simulink model "worldGenerator"  (R2016b)
settings: Solver=FixedStepAuto  StartTime=0.0  StopTime=inf  RelTol=1e-3
model workspace (MAT data in the model file):
  SL_ROS_VariableLengthArrays_MaxSizes.CommonInfo.ArrayTruncateAction = 'EmitWarning'
  SL_ROS_VariableLengthArrays_MaxSizes.MsgTypeMap = containers.Map
  SL_ROS_VariableLengthArrays_MaxSizes.MsgTypeMap.serialization.keys = {'geometry_msgs/Polygon'}
  SL_ROS_VariableLengthArrays_MaxSizes.MsgTypeMap.serialization.values{1}.PropertyName = 'Points'
  SL_ROS_VariableLengthArrays_MaxSizes.MsgTypeMap.serialization.values{1}.DataType = 'geometry_msgs/Point32'
  SL_ROS_VariableLengthArrays_MaxSizes.MsgTypeMap.serialization.values{1}.MaxLength = 32
  SL_ROS_VariableLengthArrays_MaxSizes.MsgTypeMap.serialization.uniformity = 0
  SL_ROS_VariableLengthArrays_MaxSizes.MsgTypeMap.serialization.keyType = 'char'
  SL_ROS_VariableLengthArrays_MaxSizes.MsgTypeMap.serialization.valueType = 'any'
libraries: robotlib x2
(part 1 of 2)
settings Model: Creator=jupan  LastModifiedBy=jupan
settings OptimizationCC: MaxStackSize=64
settings DebuggingCC: ParameterTunabilityLossMsg=error  FcnCallInpInsideContextMsg=warning
settings HardwareCC: ProdBitPerPointer=32  ProdBitPerSizeT=32  ProdBitPerPtrDiffT=32  ProdLargestAtomicFloat=None  ProdIntDivRoundTo=Undefined  ProdEndianess=Unspecified  ProdWordSize=32  ProdHWDeviceType=Generic->Unspecified (assume 32-bit Generic)
settings RTWCC: SystemTargetFile=ert.tlc  HardwareBoard=Robot Operating System (ROS)  TLCOptions="-aInlineSetEventsForThisBaseRateFcn=TLC_FALSE -aSuppressMultiTaskScheduler=TLC_FALSE  -aRateBasedStepFcn=0"  TemplateMakefile=ert_default_tmf  Description=Embedded Coder  GenerateReport=on  Toolchain=Catkin  IncludeHyperlinkInReport=on  LaunchReport=on  TargetLang=C++  GenerateTraceInfo=on  GenerateTraceReport=on  GenerateTraceReportSl=on  GenerateTraceReportSf=on  GenerateTraceReportEml=on
settings CodeAppCC: ForceParamTrailComments=on  IgnoreCustomStorageClasses=off  OperatorAnnotations=on  SimulinkDataObjDesc=on  SFDataObjDesc=on  MATLABFcnDesc=on  InsertBlockDesc=on  MATLABSourceComments=on
settings ERTTargetCC: SupportVariableSizeSignals=on

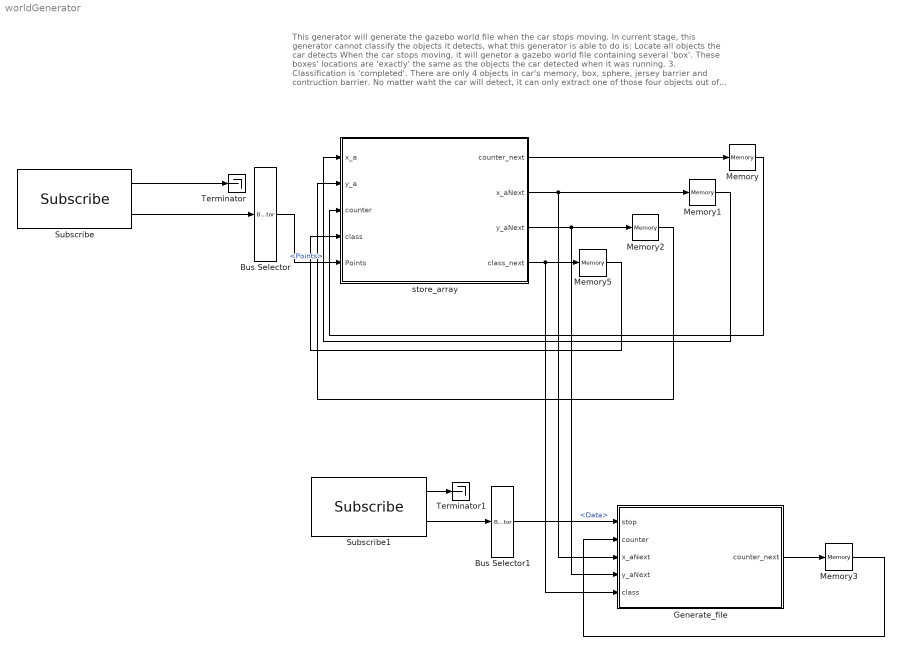
== system worldGenerator ==
  note: This generator will generate the gazebo world file when the car stops moving.
      | In current stage, this generator cannot classify the objects it detects, what this generator is able to do is:
      | Locate all objects the car detects
      | When the car stops moving, it will genetor a gazebo world file containing several 'box'.
      | These boxes' locations are 'exactly' the same as the objects the car detected when it was running.
      | 3. Classification is 'completed'. There are only 4 objects in car's memory, box, sphere, jersey barrier and contruction barrier. No matter waht the car will detect, it can only extract
      | one of those four objects out of its memory and put it into new world.
  Bus Selector : BusSelector  OutputSignals=Polygon.Points
  Bus Selector1 : BusSelector  OutputSignals=Data
  Generate_file : MATLAB Function  TreatAsAtomicUnit=on
  Memory{,1..3,5} (5 alike) : Memory
  Subscribe : robotlib/Subscribe  SourceLibraryInfo=This block requires Robotics System Toolbox  topicSource=Select from ROS network  topic=/detections  messageType=geometry_msgs/PolygonStamped  sampleTime=-1  messageQueueLength=1
  Subscribe1 : robotlib/Subscribe  SourceLibraryInfo=This block requires Robotics System Toolbox  topicSource=Specify your own  topic=/doIt  messageType=std_msgs/Bool  sampleTime=-1  messageQueueLength=1
  Terminator : Terminator
  Terminator1 : Terminator
  store_array : MATLAB Function  TreatAsAtomicUnit=on
  wires:
  Subscribe/1 -> Terminator/1
  Subscribe/2 -> Bus Selector/1
  Subscribe1/1 -> Terminator1/1
  Subscribe1/2 -> Bus Selector1/1
  store_array/1(counter_next) -> Memory/1
  store_array/2(x_aNext) -> Memory1/1, Generate_file/3(x_aNext)
  store_array/3(y_aNext) -> Memory2/1, Generate_file/4(y_aNext)
  Memory/1 -> store_array/3(counter)
  Memory1/1 -> store_array/1(x_a)
  Memory2/1 -> store_array/2(y_a)
  Bus Selector1/1 -> Generate_file/1(stop)  "<Data>"
  Generate_file/1(counter_next) -> Memory3/1
  Memory3/1 -> Generate_file/2(counter)
  store_array/4(class_next) -> Generate_file/5(class), Memory5/1
  Memory5/1 -> store_array/4(class)
  Bus Selector/1 -> store_array/5(Points)  "<Points>"

== matlab function worldGenerator/Generate_file ==
  data: stop input; counter_next output; counter input; x_aNext input; y_aNext input; class input
function counter_next = fcn(stop, counter, x_aNext, y_aNext, class)
%#codegen

if(stop && counter == 0)
    %'/home/jupan/cvchallenge_task3_ws/src/cvchallenge_task3/worlds/test.world'
    fid = fopen('gazebo_output.world', 'w+');
    % Fixed phase 1

    % <sdf version='1.4'>
    fprintf(fid, '<sdf version=''1.4''>\n');
    %   <world name='default'>
    fprintf(fid, '<world name=''default''>\n');
    %     <light name='sun' type='directional'>
    fprintf(fid, '<light name=''sun'' type=''directional''>\n');
    %       <cast_shadows>1</cast_shadows>
    fprintf(fid, '<cast_shadows>1</cast_shadows>\n');
    %       <pose>0 0 10 0 -0 0</pose>
    fprintf(fid, '<pose>0 0 10 0 -0 0</pose>\n');
    %       <diffuse>0.8 0.8 0.8 1</diffuse>
    fprintf(fid, '<diffuse>0.8 0.8 0.8 1</diffuse>\n');
    %       <specular>0.2 0.2 0.2 1</specular>
    fprintf(fid, '<specular>0.2 0.2 0.2 1</specular>\n');
    %       <attenuation>
    fprintf(fid, '<attenuation>\n');
    %         <range>1000</range>
    fprintf(fid, '<range>1000</range>\n');
    %         <constant>0.9</constant>
    fprintf(fid, '<constant>0.9</constant>\n');
    %         <linear>0.01</linear>
    fprintf(fid, '<linear>0.01</linear>\n');
    %         <quadratic>0.001</quadratic>
    fprintf(fid, '<quadratic>0.001</quadratic>\n');
    %       </attenuation>
    fprintf(fid, '</attenuation>\n');
    %       <direction>-0.5 0.1 -0.9</direction>
    fprintf(fid, '<direction>-0.5 0.1 -0.9</direction>\n');
    %     </light>
    fprintf(fid, '</light>\n');
    %     <model name='ground_plane'>
    fprintf(fid, '<model name=''ground_plane''>\n');
    %       <static>1</static>
    fprintf(fid, '<static>1</static>\n');
    %       <link name='link'>
    fprintf(fid, '<link name=''link''>\n');
    %         <collision name='collision'>
    fprintf(fid, '<collision name=''collision''>\n');
    %           <geometry>
    fprintf(fid, '<geometry>\n');
    %             <plane>
    fprintf(fid, '<plane>\n');
    %               <normal>0 0 1</normal>
    fprintf(fid, '<normal>0 0 1</normal>\n');
    %               <size>100 100</size>
    fprintf(fid, '<size>100 100</size>\n');
    %             </plane>
    fprintf(fid, '</plane>\n');
    %           </geometry>
    fprintf(fid, '</geometry>\n');
    %           <surface>
    fprintf(fid, '<surface>\n');
    %             <friction>
    fprintf(fid, '<friction>\n');
    %               <ode>
    fprintf(fid, '<ode>\n');
    %                 <mu>100</mu>
    fprintf(fid, '<mu>100</mu>\n');
    %                 <mu2>50</mu2>
    fprintf(fid, '<mu2>50</mu2>\n');
    %               </ode>
    fprintf(fid, '</ode>\n');
    %             </friction>
    fprintf(fid, '</friction>\n');
    %             <bounce/>
    fprintf(fid, '<bounce/>\n');
    %             <contact>
    fprintf(fid, '<contact>\n');
    %               <ode/>
    fprintf(fid, '<ode/>\n');
    %             </contact>
    fprintf(fid, '</contact>\n');
    %           </surface>
    fprintf(fid, '</surface>\n');
    %           <max_contacts>10</max_contacts>
    fprintf(fid, '<max_contacts>10</max_contacts>\n');
    %         </collision>
    fprintf(fid, '</collision>\n');
    %         <visual name='visual'>
    fprintf(fid, '<visual name=''visual''>\n');
    %           <cast_shadows>0</cast_shadows>
    fprintf(fid, '<cast_shadows>0</cast_shadows>\n');
    %           <geometry>
    fprintf(fid, '<geometry>\n');
    %             <plane>
    fprintf(fid, '<plane>\n');
    %               <normal>0 0 1</normal>
    fprintf(fid, '<normal>0 0 1</normal>\n');
    %               <size>100 100</size>
    fprintf(fid, '<size>100 100</size>\n');
    %             </plane>
    fprintf(fid, '</plane>\n');
    %           </geometry>
    fprintf(fid, '</geometry>\n');
    %           <material>
    fprintf(fid, '<material>\n');
    %             <script>
    fprintf(fid, '<script>\n');
    %               <uri>file://media/materials/scripts/gazebo.material</uri>
    fprintf(fid, '<uri>file://media/materials/scripts/gazebo.material</uri>\n');
    %               <name>Gazebo/Grey</name>
    fprintf(fid, '<name>Gazebo/Grey</name>\n');
    %             </script>
    fprintf(fid, '</script>\n');
    %           </material>
    fprintf(fid, '</material>\n');
    %         </visual>
    fprintf(fid, '</visual>\n');
    %         <velocity_decay>
    fprintf(fid, '<velocity_decay>\n');
    %           <linear>0</linear>
    fprintf(fid, '<linear>0</linear>\n');
    %           <angular>0</angular>
    fprintf(fid, '<angular>0</angular>\n');
    %         </velocity_decay>
    fprintf(fid, '</velocity_decay>\n');
    %         <self_collide>0</self_collide>
    fprintf(fid, '<self_collide>0</self_collide>\n');
    %         <kinematic>0</kinematic>
    fprintf(fid, '<kinematic>0</kinematic>\n');
    %         <gravity>1</gravity>
    fprintf(fid, '<gravity>1</gravity>\n');
    %       </link>
    fprintf(fid, '</link>\n');
    %     </model>
    fprintf(fid, '</model>\n');
    %     <physics type='ode'>
    fprintf(fid, '<physics type=''ode''>\n');
    %       <max_step_size>0.001</max_step_size>
    fprintf(fid, '<max_step_size>0.001</max_step_size>\n');
    %       <real_time_factor>1</real_time_factor>
    fprintf(fid, '<real_time_factor>1</real_time_factor>\n');
    %       <real_time_update_rate>1000</real_time_update_rate>
    fprintf(fid, '<real_time_update_rate>1000</real_time_update_rate>\n');
    %       <gravity>0 0 -9.8</gravity>
    fprintf(fid, '<gravity>0 0 -9.8</gravity>\n');
    %     </physics>
    fprintf(fid, '</physics>\n');
    %     <scene>
    fprintf(fid, '<scene>\n');
    %       <ambient>0.4 0.4 0.4 1</ambient>
    fprintf(fid, '<ambient>0.4 0.4 0.4 1</ambient>\n');
    %       <background>0.7 0.7 0.7 1</background>
    fprintf(fid, '<background>0.7 0.7 0.7 1</background>\n');
    %       <shadows>1</shadows>
    fprintf(fid, '<shadows>1</shadows>\n');
    %     </scene>
    fprintf(fid, '</scene>\n');
    %     <spherical_coordinates>
    fprintf(fid, '<spherical_coordinates>\n');
    %       <surface_model>EARTH_WGS84</surface_model>
    fprintf(fid, '<surface_model>EARTH_WGS84</surface_model>\n');
    %       <latitude_deg>0</latitude_deg>
    fprintf(fid, '<latitude_deg>0</latitude_deg>\n');
    %       <longitude_deg>0</longitude_deg>
    fprintf(fid, '<longitude_deg>0</longitude_deg>\n');
    %       <elevation>0</elevation>
    fprintf(fid, '<elevation>0</elevation>\n');
    %       <heading_deg>0</heading_deg>
    fprintf(fid, '<heading_deg>0</heading_deg>\n');
    %     </spherical_coordinates>
    fprintf(fid, '</spherical_coordinates>\n');
    %     <state world_name='default'>
    fprintf(fid, '<state world_name=''default''>\n');
    %       <sim_time>3437 164000000</sim_time>
    fprintf(fid, '<sim_time>3437 164000000</sim_time>\n');
    %       <real_time>3496 331503405</real_time>
    fprintf(fid, '<real_time>3496 331503405</real_time>\n');
    %       <wall_time>1490996669 500379643</wall_time>
    fprintf(fid, '<wall_time>1490996669 500379643</wall_time>\n');
    %       <model name='ground_plane'>
    fprintf(fid, '<model name=''ground_plane''>\n');
    %         <pose>0 0 0 0 -0 0</pose>
    fprintf(fid, '<pose>0 0 0 0 -0 0</pose>\n');
    %         <link name='link'>
    fprintf(fid, '<link name=''link''>\n');
    %           <pose>0 0 0 0 -0 0</pose>
    fprintf(fid, '<pose>0 0 0 0 -0 0</pose>\n');
    %           <velocity>0 0 0 0 -0 0</velocity>
    fprintf(fid, '<velocity>0 0 0 0 -0 0</velocity>\n');
    %           <acceleration>0 0 0 0 -0 0</acceleration>
    fprintf(fid, '<acceleration>0 0 0 0 -0 0</acceleration>\n');
    %           <wrench>0 0 0 0 -0 0</wrench>
    fprintf(fid, '<wrench>0 0 0 0 -0 0</wrench>\n');
    %         </link>
    fprintf(fid, '</link>\n');
    %       </model>
    fprintf(fid, '</model>\n');


    counter1 = 1;
    counter2 = 1;
    counter7 = 1;
    counter8 = 1;
    % First phase
    for i = 1:20
        if(x_aNext(i) ~= 0 && y_aNext(i) ~= 0)
            switch class(i)
              case 1 % unit_box
                  % <model name='unit_box_1'>
                  fprintf(fid, '<model name=''unit_box_');
                  fprintf(fid, '%d', int8(counter1));
                  fprintf(fid, '''>\n');
                  % <pose>-4 2 0.5 0 -0 0</pose>
                  fprintf(fid, ' <pose>');
                  fprintf(fid, '%f', x_aNext(i));fprintf(fid, ' ');
                  fprintf(fid, '%f', y_aNext(i));fprintf(fid, ' ');
                  fprintf(fid, '%f', 0.5);fprintf(fid, ' '); 
                  fprintf(fid, '%f', 0);fprintf(fid, ' ');
                  fprintf(fid, '-%f', 0);fprintf(fid, ' ');
                  fprintf(fid, '%f', 0);
                  fprintf(fid, '</pose>\n');
                  % <link name='link'>
                  fprintf(fid, ' <link name=''link''>\n');
                  % <pose>-4 2 0.5 0 -0 0</pose>
                  fprintf(fid, '  <pose>');
                  fprintf(fid, '%f', x_aNext(i));fprintf(fid, ' ');
                  fprintf(fid, '%f', y_aNext(i));fprintf(fid, ' ');
                  fprintf(fid, '%f', 0.5);fprintf(fid, ' '); 
                  fprintf(fid, '%f', 0);fprintf(fid, ' ');
                  fprintf(fid, '-%f', 0);fprintf(fid, ' ');
                  fprintf(fid, '%f', 0);
                  fprintf(fid, '</pose>\n');
                  % <velocity>0 0 0 0 -0 0</velocity>
                  fprintf(fid, '  <velocity>');
                  fprintf(fid, '%f', 0);fprintf(fid, ' ');
                  fprintf(fid, '%f', 0);fprintf(fid, ' ');
                  fprintf(fid, '%f', 0);fprintf(fid, ' '); 
                  fprintf(fid, '%f', 0);fprintf(fid, ' ');
                  fprintf(fid, '-%f', 0);fprintf(fid, ' ');
                  fprintf(fid, '%f', 0);
                  fprintf(fid, '</velocity>\n');
                  % <acceleration>0 0 0 0 -0 0</acceleration>
                  fprintf(fid, '  <acceleration>');
                  fprintf(fid, '%f', 0);fprintf(fid, ' ');
                  fprintf(fid, '%f', 0);fprintf(fid, ' ');
                  fprintf(fid, '%f', 0);fprintf(fid, ' '); 
                  fprintf(fid, '%f', 0);fprintf(fid, ' ');
                  fprintf(fid, '-%f', 0);fprintf(fid, ' ');
                  fprintf(fid, '%f', 0);
                  fprintf(fid, '</acceleration>\n');
                  % <wrench>0 0 0 0 -0 0</wrench>
                  fprintf(fid, '  <wrench>');
                  fprintf(fid, '%f', 0);fprintf(fid, ' ');
                  fprintf(fid, '%f', 0);fprintf(fid, ' ');
                  fprintf(fid, '%f', 0);fprintf(fid, ' '); 
                  fprintf(fid, '%f', 0);fprintf(fid, ' ');
                  fprintf(fid, '-%f', 0);fprintf(fid, ' ');
                  fprintf(fid, '%f', 0);
                  fprintf(fid, '</wrench>\n');
                  % </link>
                  fprintf(fid, ' </link>\n');
                  % </model>
                  fprintf(fid, '</model>\n');
                  counter1 = counter1 + 1;
              case 2 % unit_sphere
                  % <model name='unit_box_1'>
                  fprintf(fid, '<model name=''unit_sphere_');
                  fprintf(fid, '%d', int8(counter2));
                  fprintf(fid, '''>\n');
                  % <pose>-4 2 0.5 0 -0 0</pose>
                  fprintf(fid, ' <pose>');
                  fprintf(fid, '%f', x_aNext(i));fprintf(fid, ' ');
                  fprintf(fid, '%f', y_aNext(i));fprintf(fid, ' ');
                  fprintf(fid, '%f', 0.5);fprintf(fid, ' '); 
                  fprintf(fid, '%f', 0);fprintf(fid, ' ');
                  fprintf(fid, '-%f', 0);fprintf(fid, ' ');
                  fprintf(fid, '%f', 0);
                  fprintf(fid, '</pose>\n');
                  % <link name='link'>
                  fprintf(fid, ' <link name=''link''>\n');
                  % <pose>-4 2 0.5 0 -0 0</pose>
                  fprintf(fid, '  <pose>');
                  fprintf(fid, '%f', x_aNext(i));fprintf(fid, ' ');
                  fprintf(fid, '%f', y_aNext(i));fprintf(fid, ' ');
                  fprintf(fid, '%f', 0.5);fprintf(fid, ' '); 
                  fprintf(fid, '%f', 0);fprintf(fid, ' ');
                  fprintf(fid, '-%f', 0);fprintf(fid, ' ');
                  fprintf(fid, '%f', 0);
                  fprintf(fid, '</pose>\n');
                  % <velocity>0 0 0 0 -0 0</velocity>
                  fprintf(fid, '  <velocity>');
                  fprintf(fid, '%f', 0);fprintf(fid, ' ');
                  fprintf(fid, '%f', 0);fprintf(fid, ' ');
                  fprintf(fid, '%f', 0);fprintf(fid, ' '); 
                  fprintf(fid, '%f', 0);fprintf(fid, ' ');
                  fprintf(fid, '-%f', 0);fprintf(fid, ' ');
                  fprintf(fid, '%f', 0);
                  fprintf(fid, '</velocity>\n');
                  % <acceleration>0 0 0 0 -0 0</acceleration>
                  fprintf(fid, '  <acceleration>');
                  fprintf(fid, '%f', 0);fprintf(fid, ' ');
                  fprintf(fid, '%f', 0);fprintf(fid, ' ');
                  fprintf(fid, '%f', 0);fprintf(fid, ' '); 
                  fprintf(fid, '%f', 0);fprintf(fid, ' ');
                  fprintf(fid, '-%f', 0);fprintf(fid, ' ');
                  fprintf(fid, '%f', 0);
                  fprintf(fid, '</acceleration>\n');
                  % <wrench>0 0 0 0 -0 0</wrench>
                  fprintf(fid, '  <wrench>');
                  fprintf(fid, '%f', 0);fprintf(fid, ' ');
                  fprintf(fid, '%f', 0);fprintf(fid, ' ');
                  fprintf(fid, '%f', 0);fprintf(fid, ' '); 
                  fprintf(fid, '%f', 0);fprintf(fid, ' ');
                  fprintf(fid, '-%f', 0);fprintf(fid, ' ');
                  fprintf(fid, '%f', 0);
                  fprintf(fid, '</wrench>\n');
                  % </link>
                  fprintf(fid, ' </link>\n');
                  % </model>
                  fprintf(fid, '</model>\n');
                  counter2 = counter2 + 1;
                case 3
                    % <model name='unit_box_1'>
                  fprintf(fid, '<model name=''Construction Barrel_');
                  fprintf(fid, '%d', int8(counter7));
                  fprintf(fid, '''>\n');
                  % <pose>-4 2 0.5 0 -0 0</pose>
                  fprintf(fid, ' <pose>');
                  fprintf(fid, '%f', x_aNext(i));fprintf(fid, ' ');
                  fprintf(fid, '%f', y_aNext(i));fprintf(fid, ' ');
                  fprintf(fid, '%f', 0.5);fprintf(fid, ' '); 
                  fprintf(fid, '%f', 0);fprintf(fid, ' ');
                  fprintf(fid, '-%f', 0);fprintf(fid, ' ');
                  fprintf(fid, '%f', 0);
                  fprintf(fid, '</pose>\n');
                  % <link name='link'>
                  fprintf(fid, ' <link name=''link''>\n');
                  % <pose>-4 2 0.5 0 -0 0</pose>
                  fprintf(fid, '  <pose>');
                  fprintf(fid, '%f', x_aNext(i));fprintf(fid, ' ');
                  fprintf(fid, '%f', y_aNext(i));fprintf(fid, ' ');
                  fprintf(fid, '%f', 0.5);fprintf(fid, ' '); 
                  fprintf(fid, '%f', 0);fprintf(fid, ' ');
                  fprintf(fid, '-%f', 0);fprintf(fid, ' ');
                  fprintf(fid, '%f', 0);
                  fprintf(fid, '</pose>\n');
                  % <velocity>0 0 0 0 -0 0</velocity>
                  fprintf(fid, '  <velocity>');
                  fprintf(fid, '%f', 0);fprintf(fid, ' ');
                  fprintf(fid, '%f', 0);fprintf(fid, ' ');
                  fprintf(fid, '%f', 0);fprintf(fid, ' '); 
                  fprintf(fid, '%f', 0);fprintf(fid, ' ');
                  fprintf(fid, '-%f', 0);fprintf(fid, ' ');
                  fprintf(fid, '%f', 0);
                  fprintf(fid, '</velocity>\n');
                  % <acceleration>0 0 0 0 -0 0</acceleration>
                  fprintf(fid, '  <acceleration>');
                  fprintf(fid, '%f', 0);fprintf(fid, ' ');
                  fprintf(fid, '%f', 0);fprintf(fid, ' ');
                  fprintf(fid, '%f', 0);fprintf(fid, ' '); 
                  fprintf(fid, '%f', 0);fprintf(fid, ' ');
                  fprintf(fid, '-%f', 0);fprintf(fid, ' ');
                  fprintf(fid, '%f', 0);
                  fprintf(fid, '</acceleration>\n');
                  % <wrench>0 0 0 0 -0 0</wrench>
                  fprintf(fid, '  <wrench>');
                  fprintf(fid, '%f', 0);fprintf(fid, ' ');
                  fprintf(fid, '%f', 0);fprintf(fid, ' ');
                  fprintf(fid, '%f', 0);fprintf(fid, ' '); 
                  fprintf(fid, '%f', 0);fprintf(fid, ' ');
                  fprintf(fid, '-%f', 0);fprintf(fid, ' ');
                  fprintf(fid, '%f', 0);
                  fprintf(fid, '</wrench>\n');
                  % </link>
                  fprintf(fid, ' </link>\n');
                  % </model>
                  fprintf(fid, '</model>\n');
                  counter7 = counter7 + 1;
                case 4
                    % <model name='unit_box_1'>
                  fprintf(fid, '<model name=''jersey_barrier_');
                  fprintf(fid, '%d', int8(counter8));
                  fprintf(fid, '''>\n');
                  % <pose>-4 2 0.5 0 -0 0</pose>
                  fprintf(fid, ' <pose>');
                  fprintf(fid, '%f', x_aNext(i));fprintf(fid, ' ');
                  fprintf(fid, '%f', y_aNext(i));fprintf(fid, ' ');
                  fprintf(fid, '%f', 0.5);fprintf(fid, ' '); 
                  fprintf(fid, '%f', 0);fprintf(fid, ' ');
                  fprintf(fid, '-%f', 0);fprintf(fid, ' ');
                  fprintf(fid, '%f', 0);
                  fprintf(fid, '</pose>\n');
                  % <link name='link'>
                  fprintf(fid, ' <link name=''link''>\n');
                  % <pose>-4 2 0.5 0 -0 0</pose>
                  fprintf(fid, '  <pose>');
                  fprintf(fid, '%f', x_aNext(i));fprintf(fid, ' ');
                  fprintf(fid, '%f', y_aNext(i));fprintf(fid, ' ');
                  fprintf(fid, '%f', 0.5);fprintf(fid, ' '); 
                  fprintf(fid, '%f', 0);fprintf(fid, ' ');
                  fprintf(fid, '-%f', 0);fprintf(fid, ' ');
                  fprintf(fid, '%f', 0);
                  fprintf(fid, '</pose>\n');
                  % <velocity>0 0 0 0 -0 0</velocity>
                  fprintf(fid, '  <velocity>');
                  fprintf(fid, '%f', 0);fprintf(fid, ' ');
                  fprintf(fid, '%f', 0);fprintf(fid, ' ');
                  fprintf(fid, '%f', 0);fprintf(fid, ' '); 
                  fprintf(fid, '%f', 0);fprintf(fid, ' ');
                  fprintf(fid, '-%f', 0);fprintf(fid, ' ');
                  fprintf(fid, '%f', 0);
                  fprintf(fid, '</velocity>\n');
                  % <acceleration>0 0 0 0 -0 0</acceleration>
                  fprintf(fid, '  <acceleration>');
                  fprintf(fid, '%f', 0);fprintf(fid, ' ');
                  fprintf(fid, '%f', 0);fprintf(fid, ' ');
                  fprintf(fid, '%f', 0);fprintf(fid, ' '); 
                  fprintf(fid, '%f', 0);fprintf(fid, ' ');
                  fprintf(fid, '-%f', 0);fprintf(fid, ' ');
                  fprintf(fid, '%f', 0);
                  fprintf(fid, '</acceleration>\n');
                  % <wrench>0 0 0 0 -0 0</wrench>
                  fprintf(fid, '  <wrench>');
                  fprintf(fid, '%f', 0);fprintf(fid, ' ');
                  fprintf(fid, '%f', 0);fprintf(fid, ' ');
                  fprintf(fid, '%f', 0);fprintf(fid, ' '); 
                  fprintf(fid, '%f', 0);fprintf(fid, ' ');
                  fprintf(fid, '-%f', 0);fprintf(fid, ' ');
                  fprintf(fid, '%f', 0);
                  fprintf(fid, '</wrench>\n');
                  % </link>
                  fprintf(fid, ' </link>\n');
                  % </model>
                  fprintf(fid, '</model>\n');
                  counter8 = counter8 + 1;
              otherwise
                  disp('This class does not exist!') 
            end
        end
    end
    % </state>
    fprintf(fid, '</state>\n');

    counter3 = 1;
    counter4 = 1;
    counter5 = 1;
    counter6 = 1;
    % Second phase
    for j = 1:20
        if(x_aNext(j) ~= 0 && y_aNext(j) ~= 0)
            switch class(j)
              case 1 % unit_box
                  % <model name='unit_box_1'>
                  fprintf(fid, '<model name=''unit_box_');
                  fprintf(fid, '%d', int8(counter3));
                  fprintf(fid, '''>\n');
                  % <pose>-4 2 0.5 0 -0 0</pose>
                  fprintf(fid, ' <pose>');
                  fprintf(fid, '%f', x_aNext(j));fprintf(fid, ' ');
                  fprintf(fid, '%f', y_aNext(j));fprintf(fid, ' ');
                  fprintf(fid, '%f', 0.5);fprintf(fid, ' '); 
                  fprintf(fid, '%f', 0);fprintf(fid, ' ');
                  fprintf(fid, '-%f', 0);fprintf(fid, ' ');
                  fprintf(fid, '%f', 0);
                  fprintf(fid, '</pose>\n');
                  % <link name='link'>
                  fprintf(fid, ' <link name=''link''>\n');
                  % <inertial>
                  fprintf(fid, '  <inertial>\n');
                  % <mass>1</mass>
                  fprintf(fid, '   <mass>1</mass>\n');
                  % <inertia>
                  fprintf(fid, '   <inertia>\n');
                  % <ixx>1</ixx>
                  fprintf(fid, '    <ixx>1</ixx>\n');
                  fprintf(fid, '    <ixy>0</ixy>\n');
                  fprintf(fid, '    <ixz>0</ixz>\n');
                  fprintf(fid, '    <iyy>1</iyy>\n');
                  fprintf(fid, '    <iyz>0</iyz>\n');
                  fprintf(fid, '    <izz>1</izz>\n');
                  % </inertia>
                  fprintf(fid, '   </inertia>\n');
                  % </inertial>
                  fprintf(fid, '  </inertial>\n');
                  % <collision name='collision'>
                  fprintf(fid, '  <collision name=''collision''>\n');
                  % <geometry>
                  fprintf(fid, '   <geometry>\n');
                  % <box>
                  fprintf(fid, '    <box>\n');
                  % <size>1 1 1</size>
                  fprintf(fid, '     <size>');
                  fprintf(fid, '%d', int8(1));fprintf(fid, ' ');
                  fprintf(fid, '%d', int8(1));fprintf(fid, ' ');
                  fprintf(fid, '%d', int8(1));
                  fprintf(fid, '</size>\n');
                  % </box>
                  fprintf(fid, '    </box>\n');
                  % </geometry>
                  fprintf(fid, '   </geometry>\n');
                  % <max_contacts>10</max_contacts>
                  fprintf(fid, '   <max_contacts>10</max_contacts>\n');
                  % <surface>
                  fprintf(fid, '   <surface>\n');
                  % <bounce/>
                  fprintf(fid, '    <bounce/>\n');
                  % <friction>
                  fprintf(fid, '    <friction>\n');
                  % <ode/>
                  fprintf(fid, '     <ode/>\n');
                  % </friction>
                  fprintf(fid, '    </friction>\n');
                  % <contact>
                  fprintf(fid, '    <contact>\n');
                  % <ode/>
                  fprintf(fid, '     <ode/>\n');
                  % </contact>
                  fprintf(fid, '    </contact>\n');
                  % </surface>
                  fprintf(fid, '   </surface>\n');
                  % </collision>
                  fprintf(fid, '  </collision>\n');
                  % <visual name='visual'>
                  fprintf(fid, '  <visual name=''visual''>\n');
                  % <geometry>
                  fprintf(fid, '   <geometry>\n');
                  % <box>
                  fprintf(fid, '    <box>\n');
                  % <size>1 1 1</size>
                  fprintf(fid, '     <size>');
                  fprintf(fid, '%d', int8(1));fprintf(fid, ' ');
                  fprintf(fid, '%d', int8(1));fprintf(fid, ' ');
                  fprintf(fid, '%d', int8(1));
                  fprintf(fid, '</size>\n');
                  % </box>
                  fprintf(fid, '    </box>\n');
                  % </geometry>
                  fprintf(fid, '   </geometry>\n');
                  % <material>
                  fprintf(fid, '   <material>\n');
                  % <script>
                  fprintf(fid, '    <script>\n');
                  % <uri>file://media/materials/scripts/gazebo.material</uri>
                  fprintf(fid, '     <uri>file://media/materials/scripts/gazebo.material</uri>\n');
                  % <name>Gazebo/Grey</name>
                  fprintf(fid, '     <name>Gazebo/Grey</name>\n');
                  % </script>
                  fprintf(fid, '    </script>\n');
                  % </material>
                  fprintf(fid, '   </material>\n');
                  % </visual>
                  fprintf(fid, '  </visual>\n');
                  % <velocity_decay>
                  fprintf(fid, '  <velocity_decay>\n');
                  % <linear>0</linear>
                  fprintf(fid, '   <linear>0</linear>\n');
                  % <angular>0</angular>
                  fprintf(fid, '   <angular>0</angular>\n');
                  % </velocity_decay>
                  fprintf(fid, '  </velocity_decay>\n');
                  % <self_collide>0</self_collide>
                  fprintf(fid, '  <self_collide>0</self_collide>\n');
                  % <kinematic>0</kinematic>
                  fprintf(fid, '  <kinematic>0</kinematic>\n');
                  % <gravity>1</gravity>
                  fprintf(fid, '  <gravity>1</gravity>\n');
                  % </link>
                  fprintf(fid, ' </link>\n');
                  % <static>0</static>
                  fprintf(fid, ' <static>0</static>\n');
                  % </model>
                  fprintf(fid, '</model>\n');
                  counter3 = counter3 + 1;
              case 2 % unit_sphere
                  % <model name='unit_sphere_1'>
                  fprintf(fid, '<model name=''unit_sphere_');
                  fprintf(fid, '%d', int8(counter4));
                  fprintf(fid, '''>\n');
                  % <pose>-4 2 0.5 0 -0 0</pose>
                  fprintf(fid, ' <pose>');
                  fprintf(fid, '%f', x_aNext(j));fprintf(fid, ' ');
                  fprintf(fid, '%f', y_aNext(j));fprintf(fid, ' ');
                  fprintf(fid, '%f', 0.5);fprintf(fid, ' '); 
                  fprintf(fid, '%f', 0);fprintf(fid, ' ');
                  fprintf(fid, '-%f', 0);fprintf(fid, ' ');
                  fprintf(fid, '%f', 0);
                  fprintf(fid, '</pose>\n');
                  % <link name='link'>
                  fprintf(fid, ' <link name=''link''>\n');
                  % <inertial>
                  fprintf(fid, '  <inertial>\n');
                  % <mass>1</mass>
                  fprintf(fid, '   <mass>1</mass>\n');
                  % <inertia>
                  fprintf(fid, '   <inertia>\n');
                  % <ixx>1</ixx>
                  fprintf(fid, '    <ixx>1</ixx>\n');
                  fprintf(fid, '    <ixy>0</ixy>\n');
                  fprintf(fid, '    <ixz>0</ixz>\n');
                  fprintf(fid, '    <iyy>1</iyy>\n');
                  fprintf(fid, '    <iyz>0</iyz>\n');
                  fprintf(fid, '    <izz>1</izz>\n');
                  % </inertia>
                  fprintf(fid, '   </inertia>\n');
                  % </inertial>
                  fprintf(fid, '  </inertial>\n');
                  % <collision name='collision'>
                  fprintf(fid, '  <collision name=''collision''>\n');
                  % <geometry>
                  fprintf(fid, '   <geometry>\n');
                  % <box>
                  fprintf(fid, '    <sphere>\n');
                  % <size>1 1 1</size>
                  fprintf(fid, '    <radius>0.5</radius>\n');
                  % </box>
                  fprintf(fid, '    </sphere>\n');
                  % </geometry>
                  fprintf(fid, '   </geometry>\n');
                  % <max_contacts>10</max_contacts>
                  fprintf(fid, '   <max_contacts>10</max_contacts>\n');
                  % <surface>
                  fprintf(fid, '   <surface>\n');
                  % <bounce/>
                  fprintf(fid, '    <bounce/>\n');
                  % <friction>
                  fprintf(fid, '    <friction>\n');
                  % <ode/>
                  fprintf(fid, '     <ode/>\n');
                  % </friction>
                  fprintf(fid, '    </friction>\n');
                  % <contact>
                  fprintf(fid, '    <contact>\n');
                  % <ode/>
                  fprintf(fid, '     <ode/>\n');
                  % </contact>
                  fprintf(fid, '    </contact>\n');
                  % </surface>
                  fprintf(fid, '   </surface>\n');
                  % </collision>
                  fprintf(fid, '  </collision>\n');
                  % <visual name='visual'>
                  fprintf(fid, '  <visual name=''visual''>\n');
                  % <geometry>
                  fprintf(fid, '   <geometry>\n');
                  % <sphere>
                  fprintf(fid, '    <sphere>\n');
                  % <radius>0.5</radius>
                  fprintf(fid, '     <radius>0.5</radius>\n');
                  % </sphere>
                  fprintf(fid, '    </sphere>\n');
                  % </geometry>
                  fprintf(fid, '   </geometry>\n');
                  % <material>
                  fprintf(fid, '   <material>\n');
                  % <script>
                  fprintf(fid, '    <script>\n');
                  % <uri>file://media/materials/scripts/gazebo.material</uri>
                  fprintf(fid, '     <uri>file://media/materials/scripts/gazebo.material</uri>\n');
                  % <name>Gazebo/Grey</name>
                  fprintf(fid, '     <name>Gazebo/Grey</name>\n');
                  % </script>
                  fprintf(fid, '    </script>\n');
                  % </material>
                  fprintf(fid, '   </material>\n');
                  % </visual>
                  fprintf(fid, '  </visual>\n');
                  % <velocity_decay>
                  fprintf(fid, '  <velocity_decay>\n');
                  % <linear>0</linear>
                  fprintf(fid, '   <linear>0</linear>\n');
                  % <angular>0</angular>
                  fprintf(fid, '   <angular>0</angular>\n');
                  % </velocity_decay>
                  fprintf(fid, '  </velocity_decay>\n');
                  % <self_collide>0</self_collide>
                  fprintf(fid, '  <self_collide>0</self_collide>\n');
                  % <kinematic>0</kinematic>
                  fprintf(fid, '  <kinematic>0</kinematic>\n');
                  % <gravity>1</gravity>
                  fprintf(fid, '  <gravity>1</gravity>\n');
                  % </link>
                  fprintf(fid, ' </link>\n');
                  % <static>0</static>
                  fprintf(fid, ' <static>0</static>\n');
                  % </model>
                  fprintf(fid, '</model>\n');
                  counter4 = counter4 + 1;
                case 3
                    % Construction Barrel
                    fprintf(fid, '<model name=''Construction Barrel_');
                              fprintf(fid, '%d', int8(counter5));
                              fprintf(fid, '''>\n');
                    fprintf(fid, ['<link name=''link''>\n'...
                            ,'<inertial>\n'...
                             , '<pose>0 0 0.4 0 -0 0</pose>\n'...
                              ,'<mass>500</mass>\n'...
                              ,'<inertia>\n'...
                                ,'<ixx>51.2096</ixx>\n'...
                                ,'<iyy>51.2096</iyy>\n'...
                                ,'<izz>25</izz>\n'...
                                ,'<ixy>0</ixy>\n'...
                                ,'<ixz>0</ixz>\n'...
                                ,'<iyz>0</iyz>\n'...
                              ,'</inertia>\n'...
                            ,'</inertial>\n'...
                            ,'<collision name=''collision''>\n'...
                              ,'<geometry>\n'...
                                ,'<mesh>\n'...
                                  ,'<uri>model://construction_barrel/meshes/construction_barrel.dae</uri>\n'...
                                ,'</mesh>\n'...
                              ,'</geometry>\n'...
                              ,'<max_contacts>10</max_contacts>\n'...
                              ,'<surface>\n'...
                                ,'<bounce/>\n'...
                                ,'<friction>\n'...
                                  ,'<ode/>\n'...
                                ,'</friction>\n'...
                                ,'<contact>\n'...
                                  ,'<ode/>\n'...
                                ,'</contact>\n'...
                              ,'</surface>\n'...
                            ,'</collision>\n'...
                            ,'<visual name=''visual''>\n'...
                              ,'<geometry>\n'...
                                ,'<mesh>\n'...
                                  ,'<uri>model://construction_barrel/meshes/construction_barrel.dae</uri>\n'...
                                ,'</mesh>\n'...
                              ,'</geometry>\n'...
                            ,'</visual>\n'...
                            ,'<velocity_decay>\n'...
                              ,'<linear>0</linear>\n'...
                              ,'<angular>0</angular>\n'...
                            ,'</velocity_decay>\n'...
                            ,'<self_collide>0</self_collide>\n'...
                            ,'<kinematic>0</kinematic>\n'...
                            ,'<gravity>1</gravity>\n'...
                          ,'</link>\n']);
                      fprintf(fid, ' <pose>');
                          fprintf(fid, '%f', x_aNext(j));fprintf(fid, ' ');
                          fprintf(fid, '%f', y_aNext(j));fprintf(fid, ' ');
                          fprintf(fid, '%f', 0.5);fprintf(fid, ' '); 
                          fprintf(fid, '%f', 0);fprintf(fid, ' ');
                          fprintf(fid, '-%f', 0);fprintf(fid, ' ');
                          fprintf(fid, '%f', 0);
                          fprintf(fid, '</pose>\n');
                     fprintf(fid, ['<static>0</static>\n'...
                    ,'</model>\n']);
                     counter5 = counter5 + 1;
                case 4
                    % jersey barrier
                    fprintf(fid, '<model name=''jersey_barrier_');
                              fprintf(fid, '%d', int8(counter6));
                              fprintf(fid, '''>\n');
                    fprintf(fid, ['<static>1</static>\n'...
                          ,'<link name=''link''>\n'...
                            ,'<visual name=''visual''>\n'...
                             ,'<geometry>\n'...
                                ,'<mesh>\n'...
                                  ,'<uri>model://jersey_barrier/meshes/jersey_barrier.dae</uri>\n'...
                                ,'</mesh>\n'...
                              ,'</geometry>\n'...
                            ,'</visual>\n'...
                            ,'<collision name=''upright''>\n'...
                              ,'<pose>0 0 0.5715 0 -0 0</pose>\n'...
                              ,'<geometry>\n'...
                                ,'<box>\n'...
                                  ,'<size>4.06542 0.3063 1.143</size>\n'...
                                ,'</box>\n'...
                              ,'</geometry>\n'...
                              ,'<max_contacts>10</max_contacts>\n'...
                              ,'<surface>\n'...
                                ,'<bounce/>\n'...
                                ,'<friction>\n'...
                                  ,'<ode/>\n'...
                                ,'</friction>\n'...
                                ,'<contact>\n'...
                                  ,'<ode/>\n'...
                                ,'</contact>\n'...
                              ,'</surface>\n'...
                            ,'</collision>\n'...
                            ,'<collision name=''base''>\n'...
                              ,'<pose>0 0 0.032258 0 -0 0</pose>\n'...
                              ,'<geometry>\n'...
                                ,'<box>\n'...
                                  ,'<size>4.06542 0.8107 0.064516</size>\n'...
                                ,'</box>\n'...
                              ,'</geometry>\n'...
                              ,'<max_contacts>10</max_contacts>\n'...
                              ,'<surface>\n'...
                                ,'<bounce/>\n'...
                                ,'<friction>\n'...
                                  ,'<ode/>\n'...
                                ,'</friction>\n'...
                                ,'<contact>\n'...
                                  ,'<ode/>\n'...
                                ,'</contact>\n'...
                              ,'</surface>\n'...
                            ,'</collision>\n'...
                            ,'<collision name=''base2''>\n'...
                              ,'<pose>0 0 0.1 0 -0 0</pose>\n'...
                              ,'<geometry>\n'...
                                ,'<box>\n'...
                                  ,'<size>4.06542 0.65 0.1</size>\n'...
                                ,'</box>\n'...
                              ,'</geometry>\n'...
                              ,'<max_contacts>10</max_contacts>\n'...
                              ,'<surface>\n'...
                                ,'<bounce/>\n'...
                                ,'<friction>\n'...
                                  ,'<ode/>\n'...
                                ,'</friction>\n'...
                                ,'<contact>\n'...
                                  ,'<ode/>\n'...
                                ,'</contact>\n'...
                              ,'</surface>\n'...
                            ,'</collision>\n'...
                            ,'<collision name=''base3''>\n'...
                              ,'<pose>0 0 0.2 0 -0 0</pose>\n'...
                              ,'<geometry>\n'...
                                ,'<box>\n'...
                                  ,'<size>4.06542 0.5 0.1</size>\n'...
                                ,'</box>\n'...
                              ,'</geometry>\n'...
                              ,'<max_contacts>10</max_contacts>\n'...
                              ,'<surface>\n'...
                                ,'<bounce/>\n'...
                                ,'<friction>\n'...
                                  ,'<ode/>\n'...
                                ,'</friction>\n'...
                                ,'<contact>\n'...
                                  ,'<ode/>\n'...
                                ,'</contact>\n'...
                              ,'</surface>\n'...
                            ,'</collision>\n'...
                            ,'<collision name=''left-angle''>\n'...
                              ,'<pose>0 -0.224 0.2401 0.9 -0 0</pose>\n'...
                              ,'<geometry>\n'...
                                ,'<box>\n'...
                                  ,'<size>4.06542 0.5 0.064516</size>\n'...
                                ,'</box>\n'...
                              ,'</geometry>\n'...
                              ,'<max_contacts>10</max_contacts>\n'...
                              ,'<surface>\n'...
                                ,'<bounce/>\n'...
                                ,'<friction>\n'...
                                  ,'<ode/>\n'...
                                ,'</friction>\n'...
                                ,'<contact>\n'...
                                  ,'<ode/>\n'...
                                ,'</contact>\n'...
                              ,'</surface>\n'...
                            ,'</collision>\n'...
                            ,'<collision name=''right-angle''>\n'...
                              ,'<pose>0 0.224 0.2401 -0.9 0 0</pose>\n'...
                              ,'<geometry>\n'...
                                ,'<box>\n'...
                                  ,'<size>4.06542 0.5 0.064516</size>\n'...
                                ,'</box>\n'...
                              ,'</geometry>\n'...
                              ,'<max_contacts>10</max_contacts>\n'...
                              ,'<surface>\n'...
                                ,'<bounce/>\n'...
                                ,'<friction>\n'...
                                  ,'<ode/>\n'...
                                ,'</friction>\n'...
                                ,'<contact>\n'...
                                  ,'<ode/>\n'...
                                ,'</contact>\n'...
                              ,'</surface>\n'...
                            ,'</collision>\n'...
                            ,'<velocity_decay>\n'...
                              ,'<linear>0</linear>\n'...
                              ,'<angular>0</angular>\n'...
                            ,'</velocity_decay>\n'...
                            ,'<self_collide>0</self_collide>\n'...
                            ,'<kinematic>0</kinematic>\n'...
                            ,'<gravity>1</gravity>\n'...
                          ,'</link>\n']);
                         fprintf(fid, ' <pose>');
                              fprintf(fid, '%f', x_aNext(j));fprintf(fid, ' ');
                              fprintf(fid, '%f', y_aNext(j));fprintf(fid, ' ');
                              fprintf(fid, '%f', 0.5);fprintf(fid, ' '); 
                              fprintf(fid, '%f', 0);fprintf(fid, ' ');
                              fprintf(fid, '-%f', 0);fprintf(fid, ' ');
                              fprintf(fid, '%f', 0);
                              fprintf(fid, '</pose>\n');
                         fprintf(fid, ['</model>\n']);
                         counter6 = counter6 + 1;
              otherwise
                  disp('This class does not exist!') 
            end
        end
    end

    % Fixed phase 2

    % <gui fullscreen='0'>
    fprintf(fid, '<gui fullscreen=''0''>\n');
    %       <camera name='user_camera'>
    fprintf(fid, '<camera name=''user_camera''>\n');
    %         <pose>26.0416 -23.4949 28.141 3.53447e-17 0.667643 2.38819</pose>
    fprintf(fid, '<pose>26.0416 -23.4949 28.141 3.53447e-17 0.667643 2.38819</pose>\n');
    %         <view_controller>orbit</view_controller>
    fprintf(fid, '<view_controller>orbit</view_controller>\n');
    %       </camera>
    fprintf(fid, '</camera>\n');
    %     </gui>
    fprintf(fid, '</gui>\n');
    %   </world>
    fprintf(fid, '</world>\n');
    % </sdf>
    fprintf(fid, '</sdf>\n');

    fclose('all');
    
    counter = 1;
    counter_next = counter;
elseif(~stop)
    counter_next = 0;
else
    counter_next = 1;
end
